simulink model "CITRIS"  (Simulink 7.4)
settings: Solver=FixedStepDiscrete  StartTime=0.0  StopTime=20  FixedStep=1  MaxStep=1  RelTol=1e-3
values from neighbouring files (symbols this model uses):
  mdot = [mdot controlInputHistory{i}(1,:)']    [CITRISBLOMSimulation.m]
  mdotmax = 740    [CITRISBLOMSimulation.m]
  mdotmin = 220    [CITRISBLOMSimulation.m]
  model =     [model.mat]
  T0 = 21    [CITRISBLOMSimulation.m]
  vlv = [vlv controlInputHistory{i}(2,:)']    [CITRISBLOMSimulation.m]
undefined symbols (not defined in the file or in its folder): i, mdotTk, mdotvlv, mdotvlvk, Tk, TmaxSlack, TmaxV, TminSlack, TminV, wk, wk_1, wk_2
libraries: BLOM_Lib x18
settings Model: Creator=vichik  LastModifiedBy=Kyle
settings OptimizationCC: InitFltsAndDblsToZero=on

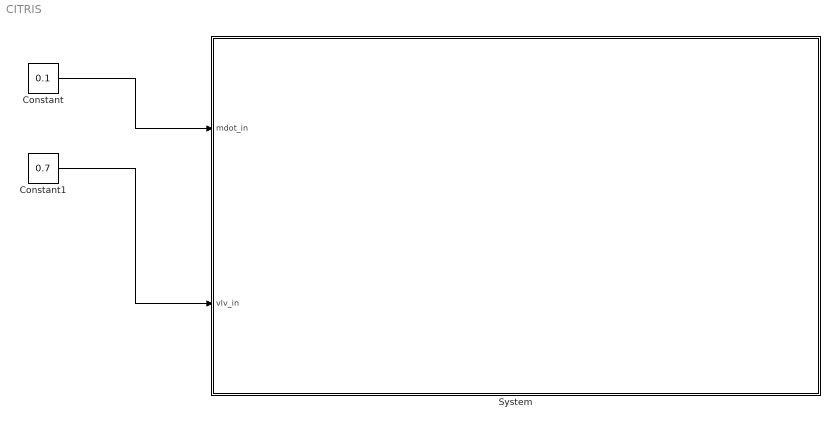
== system CITRIS ==
  Constant : Constant  Value=0.1
  Constant1 : Constant  Value=0.7
  System : Subsystem
  wires:
  Constant/1 -> System/1(mdot_in)
  Constant1/1 -> System/2(vlv_in)

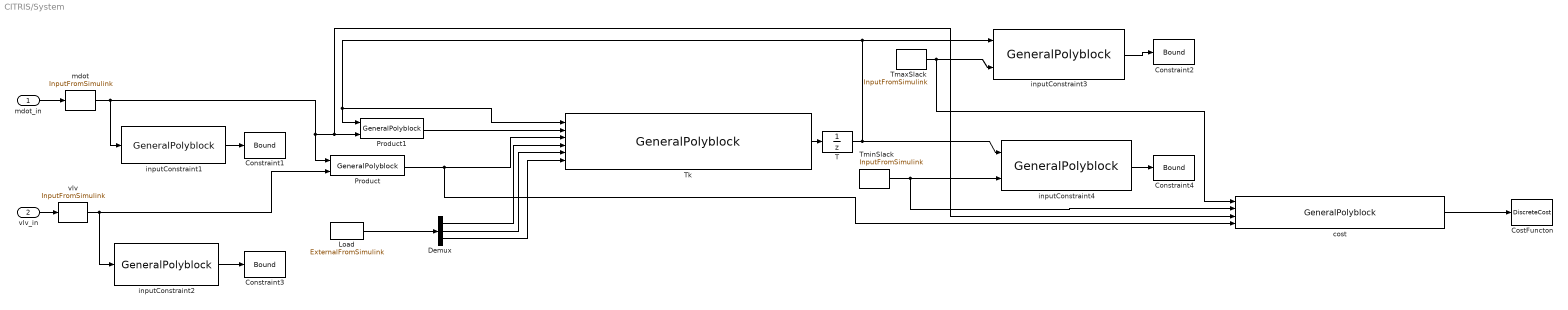
== system CITRIS/System ==
  mdot_in : Inport
  vlv_in : Inport  Port=2
  Constraint{1..4} (4 alike) : BLOM_Lib/Bound  SystemSampleTime=-1  ub=0  lb=-inf  initial_step=on  final_step=on  intermediate_step=on
  CostFuncton : BLOM_Lib/DiscreteCost  SystemSampleTime=-1  initial_step=on  final_step=on  intermediate_step=on
  Demux : Demux  Outputs=3
  Load : BLOM_Lib/ExternalFromSimulink  SystemSampleTime=-1  interpType=Zero-Order Hold
  Product : BLOM_Lib/GeneralPolyblock  SystemSampleTime=-1  P_f="[1  1  ]"  K_f=[1 ]  P_g=[0 0]  K_g=1  inputs=mdot,vlv  inputScalar=on  outputScalar=on
  Product1 : BLOM_Lib/GeneralPolyblock  SystemSampleTime=-1  P_f="[1  1  ]"  K_f=[1 ]  P_g=[0 0]  K_g=1  inputs=Tk,mdot  inputScalar=on  outputScalar=on
  T : UnitDelay  X0=T0  SampleTime=-1
  Tk : BLOM_Lib/GeneralPolyblock  SystemSampleTime=-1  P_f=[1 0 0 0 0 0;0 1 0 0 0 0;0 0 1 0 0 0;0 0 0 1 0 0;0 0 0 0 1 0;0 0 0 0 0 1;0 0 0 0 0 0]  K_f=[model{i}.A model{i}.B2 model{i}.B1 model{i}.W(1) model{i}.W(2) model{i}.W(3) model{i}.C]  P_g=[0 0 0 0 0 0]  K_g=1  inputs=Tk,mdotTk,mdotvlvk,wk,wk_1,wk_2  inputScalar=on  outputScalar=on
  TmaxSlack : BLOM_Lib/InputFromSimulink  SystemSampleTime=-1  interpType=Zero-Order Hold
  TminSlack : BLOM_Lib/InputFromSimulink  SystemSampleTime=-1  interpType=Zero-Order Hold
  cost : BLOM_Lib/GeneralPolyblock  SystemSampleTime=-1  P_f=[1 0 0 0;0 1 0 0;0 0 2 0;0 0 0 1]  K_f=[10 10 0.7*1e-6 1e-5]  P_g=[0 0 0 0]  K_g=1  inputs=TmaxV,TminV,mdot,mdotvlv  inputScalar=on  outputScalar=on
  inputConstraint1 : BLOM_Lib/GeneralPolyblock  SystemSampleTime=-1  P_f="[1  ;  0 ]"  K_f=[1 -mdotmax; -1 mdotmin]  P_g="[0  ]"  K_g=1  inputs=mdot  inputScalar=on  outputScalar=off
  inputConstraint2 : BLOM_Lib/GeneralPolyblock  SystemSampleTime=-1  P_f=[1;0]  K_f="[1 -100; -1  0]"  P_g=[0]  K_g=1  inputs=vlv  inputScalar=on  outputScalar=off
  inputConstraint3 : BLOM_Lib/GeneralPolyblock  SystemSampleTime=-1  P_f=[1 0;0 1;0 0]  K_f=[1 -1 -22;0 -1 0]  P_g=[0 0]  K_g=1  inputs=Tk,TmaxSlack  inputScalar=on  outputScalar=off
  inputConstraint4 : BLOM_Lib/GeneralPolyblock  SystemSampleTime=-1  P_f=[1 0;0 1;0 0]  K_f=[-1 -1 20;0 -1 0]  P_g=[0 0]  K_g=1  inputs=Tk,TminSlack  inputScalar=on  outputScalar=off
  mdot : BLOM_Lib/InputFromSimulink  SystemSampleTime=-1  interpType=Zero-Order Hold
  vlv : BLOM_Lib/InputFromSimulink  SystemSampleTime=-1  interpType=Zero-Order Hold
  wires:
  T/1 -> inputConstraint3/1, Product1/1, Tk/1, inputConstraint4/1
  mdot/1 -> cost/3, Product1/2, Product/1, inputConstraint1/1
  cost/1 -> CostFuncton/1
  mdot_in/1 -> mdot/1
  inputConstraint1/1 -> Constraint1/1
  vlv_in/1 -> vlv/1
  vlv/1 -> Product/2, inputConstraint2/1
  inputConstraint2/1 -> Constraint3/1
  Load/1 -> Demux/1
  Demux/1 -> Tk/4
  Demux/2 -> Tk/5
  Demux/3 -> Tk/6
  Product1/1 -> Tk/2
  Product/1 -> cost/4, Tk/3
  inputConstraint3/1 -> Constraint2/1
  TmaxSlack/1 -> cost/1, inputConstraint3/2
  inputConstraint4/1 -> Constraint4/1
  TminSlack/1 -> cost/2, inputConstraint4/2
  Tk/1 -> T/1
